simulink model "sldemo_mdlref_dsm"  (R2017b)
settings: Solver=FixedStepDiscrete  StartTime=0.0  StopTime=10.0  FixedStep=0.1  RelTol=1e-3  EnableMultiTasking=on
PreLoadFcn:
  | load sldemo_mdlref_dsm_data.mat
Description:
  | Model Reference and Global Data Stores
  | 
  | This example explains how to define and use global data stores to
  | share global data among reference models.
settings Model: ModifiedByFormat=The MathWorks Inc.  ExtModeAutoUpdateStatusClock=off  Creator=The MathWorks, Inc.  LastModifiedBy=The MathWorks Inc.
settings DataIOCC: LimitDataPoints=on  SaveFormat=Array
settings OptimizationCC: DefaultParameterBehavior=Inlined  ExpressionDepthLimit=2147483647  InitFltsAndDblsToZero=on  LifeSpan=inf
settings DebuggingCC: SaveWithParameterizedLinksMsg=none  UnderspecifiedInitializationDetection=Classic  MergeDetectMultiDrivingBlocksExec=none  SolverPrmCheckMsg=warning  MultiTaskCondExecSysMsg=none  SigSpecEnsureSampleTimeMsg=none  FcnCallInpInsideContextMsg=warning  BusObjectLabelMismatch=error  RootOutportRequireBusObject=error  StateNameClashWarn=warning  StrictBusMsg=ErrorOnBusTreatedAsVector  SFUnexpectedBacktrackingDiag=warning  SFNoUnconditionalDefaultTransitionDiag=warning  SFExecutionAtInitializationDiag=none
settings HardwareCC: ProdBitPerPointer=32  ProdBitPerSizeT=32  ProdBitPerPtrDiffT=32  ProdLargestAtomicFloat=None  ProdIntDivRoundTo=Undefined  ProdEndianess=Unspecified  ProdWordSize=32  ProdHWDeviceType=32-bit Generic
settings ModelReferenceCC: UpdateModelReferenceTargets=IfOutOfDate  PropagateSignalLabelsOutOfModel=off
settings RTWCC: Description=Generic Real-Time Target
settings CodeAppCC: MaxIdLength=100  StateflowObjectComments=on
settings GRTTargetCC: TargetFcnLib=ansi_tfl_tmw.mat  TargetLangStandard=C89/C90 (ANSI)  GeneratePreprocessorConditionals=Disable all  CombineOutputUpdateFcns=off  GRTInterface=on
settings ConfigComp: CovMetricSettings=dw  CovHtmlReporting=on  CovSaveCumulativeToWorkspaceVar=on  CovSaveSingleToWorkspaceVar=on  CovExternalEMLEnable=off  CovSFcnEnable=off

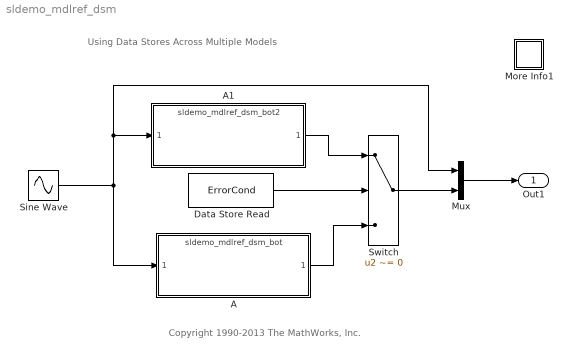
== system sldemo_mdlref_dsm ==
  note: Copyright 1990-2013 The MathWorks, Inc.
  note: Using Data Stores Across Multiple Models
  A : ModelReference  ModelNameDialog=sldemo_mdlref_dsm_bot  SimulationMode=Normal  ModelReferenceVersion=1.55
  A1 : ModelReference  ModelNameDialog=sldemo_mdlref_dsm_bot2  SimulationMode=Normal  ModelReferenceVersion=1.36
  Data Store Read : DataStoreRead  DataStoreName=ErrorCond  SampleTime=0.1
  More Info1 : Subsystem
      settings: OpenFcn=showdemo(bdroot(gcb))
      mask Display: disp('?')
  Mux : Mux  Inputs=2
  Sine Wave : Sin  SampleTime=0.1
  Switch : Switch  Criteria=u2 ~= 0
  Out1 : Outport
  wires:
  Sine Wave/1 -> Mux/1, A1/1, A/1
  Data Store Read/1 -> Switch/2
  Switch/1 -> Mux/2
  Mux/1 -> Out1/1
  A1/1 -> Switch/1
  A/1 -> Switch/3

== system sldemo_mdlref_dsm/More Info1 ==
